simulink model "quad"  (R2018b)
settings: Solver=VariableStepAuto  StartTime=0.0  StopTime=100  RelTol=1e-3  EnableMultiTasking=on
InitFcn:
  | %%Motor
  | fs_servo = 50; %Hz
  | Ts_servo = 1/fs_servo;
  | rate = 1200; % rad/s per second change
  | limit = 1200; % rad/s
  | 
  | %%Controller
  | fs = 200; % Hz
  | Ts = 1/fs;
  | 
  | g = 9.81; % Gravity
values from neighbouring files (symbols this model uses):
  F = zeros(3, numPoints)    [test_cyclorotor.m]
  r = 0.069    [Cyclorotor.m]
undefined symbols (not defined in the file or in its folder): MIL
libraries: simulink x13, aerolibwind2 x1, sharedtransform x1
settings Model: Creator=fs349  LastModifiedBy=Jamie
settings DataIOCC: SaveState=on
settings OptimizationCC: LifeSpan=inf
settings DebuggingCC: AllowSymbolicDim=off  SFUnexpectedBacktrackingDiag=warning  SFNoUnconditionalDefaultTransitionDiag=warning  SFExecutionAtInitializationDiag=none
settings ModelReferenceCC: PropagateSignalLabelsOutOfModel=off
settings SFSimCC: SimUseLocalCustomCode=off
settings RTWCC: RTWUseLocalCustomCode=off
settings CodeAppCC: StateflowObjectComments=on
settings GRTTargetCC: TargetLangStandard=C89/C90 (ANSI)
settings ConfigComp: CovMetricSettings=dw  CovHtmlReporting=on  CovSaveCumulativeToWorkspaceVar=on  CovSaveSingleToWorkspaceVar=on  CovExternalEMLEnable=off

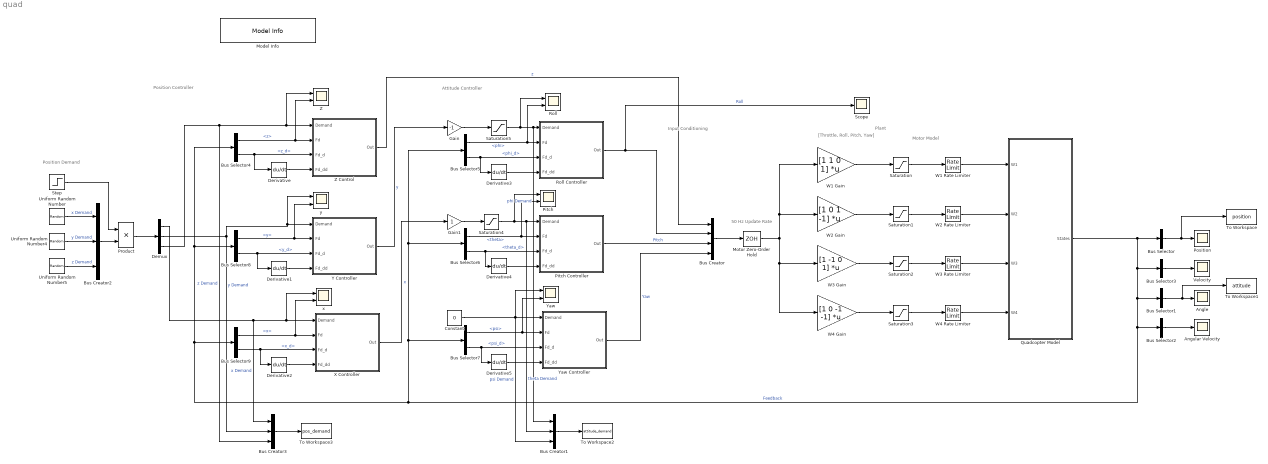
== system quad ==
  note: 50 Hz Update Rate
  note: Position Controller
  note: Attitude Controller
  note: Motor Model
  note: Plant
  note: Input Conditioning
  note: [Throttle, Roll, Pitch, Yaw]
  note: Position Demand
  Angle : Scope
  Angular Velocity : Scope
  Bus Creator : BusCreator  Inputs=4
  Bus Creator1 : BusCreator  Inputs=3
  Bus Creator2 : BusCreator  Inputs=3
  Bus Creator3 : BusCreator  Inputs=3
  Bus Selector : BusSelector  OutputSignals=x,y,z  OutputAsBus=on
  Bus Selector1 : BusSelector  OutputSignals=phi,theta,psi  OutputAsBus=on
  Bus Selector2 : BusSelector  OutputSignals=phi_d,theta_d,psi_d  OutputAsBus=on
  Bus Selector3 : BusSelector  OutputSignals=x_d,y_d,z_d  OutputAsBus=on
  Bus Selector4 : BusSelector  OutputSignals=z,z_d
  Bus Selector5 : BusSelector  OutputSignals=phi,phi_d
  Bus Selector6 : BusSelector  OutputSignals=theta,theta_d
  Bus Selector7 : BusSelector  OutputSignals=psi,psi_d
  Bus Selector8 : BusSelector  OutputSignals=y,y_d
  Bus Selector9 : BusSelector  OutputSignals=x,x_d
  Constant : Constant  Value=0
  Demux : Demux  Outputs=3
  Derivative{,1..5} (6 alike) : Derivative
  Gain : Gain  Gain=-1
  Gain1 : Gain
  Model Info : simulink/Model-Wide Utilities/Model Info  Frame=on  DisplayStringWithTags=|  HorizontalTextAlignment=Left  LeftAlignmentValue=0.02
      | Last Modified: %<ModifiedDate>
      | By: %<LastModifiedBy>
      | version: %<ModelVersion>
  Motor Zero-Order Hold : ZeroOrderHold  SampleTime=Ts_servo
  Pitch : Scope  NumInputPorts=2
  Pitch Controller : Subsystem  mask{P1=6, I1=0, D1=5, P2=1, I2=0, D2=0.03}
      mask prompts: P1 "P1, Proportional"; I1 "I1, Integral"; D1 "D1, Derivative"; P2 "P2, Proportional"; I2 "I2, Integral"; D2 "D2, Derivative"
      mask DialogControl Container3 Prompt: Outer Loop
      mask DialogControl Container4 Prompt: Inner Loop
  Position : Scope
  Product : Product
  Quadcopter Model : Subsystem  mask{g=g, m=0.468, k=2.98e-6, Ixx=4.856e-3, Iyy=4.856e-3, Izz=8.801e-3, b=1.14e-7, L=0.225, Ax=0.25, Ay=0.25, Az=0.25, ws=4.5}
      mask prompts: g "g, Gravity (m/s^2)"; m "m, Quad mass (kg)"; k "k, Angular velocity thrust proportional constant"; Ixx "Ixx, x inertia (kg m^2)"; Iyy "Iyy, y inertia (kg m^2)"; Izz "Izz, z intertia (kg m^2)"; b "b, Yaw torque angular velocity proportional constant"; L "L, Arm length (m)"; Ax "Ax, x drag Coefficient"; Ay "Ay, y drag Coefficien"; Az "Az, z drag Coefficien"; ws "ws, Wind Speed"
      mask DialogControl Container4 Prompt: Quad Properties
      mask DialogControl Container5 Prompt: Modelling Properies
  Roll : Scope  NumInputPorts=2
  Roll Controller : Subsystem  mask{P1=6, I1=0, D1=5, P2=1, I2=0, D2=0.03}
      mask prompts: P1 "P1, Proportional"; I1 "I1, Integral"; D1 "D1, Derivative"; P2 "P2, Proportional"; I2 "I2, Integral"; D2 "D2, Derivative"
      mask DialogControl Container3 Prompt: Outer Loop
      mask DialogControl Container4 Prompt: Inner Loop
  Saturation{,1..3} (4 alike) : Saturate  UpperLimit=limit  LowerLimit=0
  Saturation4 : Saturate  UpperLimit=pi/3  LowerLimit=-pi/3
  Saturation5 : Saturate  UpperLimit=pi/3  LowerLimit=-pi/3
  Scope : Scope
  Step : Step  Time=20  SampleTime=0
  To Workspace : ToWorkspace  VariableName=position  SaveFormat=Timeseries  SampleTime=-1
  To Workspace1 : ToWorkspace  VariableName=attitude  SaveFormat=Timeseries  SampleTime=-1
  To Workspace2 : ToWorkspace  VariableName=attitude_demand  SaveFormat=Timeseries  SampleTime=-1
  To Workspace3 : ToWorkspace  VariableName=pos_demand  SaveFormat=Timeseries  SampleTime=-1
  Uniform Random Number : UniformRandomNumber  Minimum=-3  Maximum=3  SampleTime=10
  Uniform Random Number4 : UniformRandomNumber  Minimum=-3  Maximum=3  Seed=1  SampleTime=10
  Uniform Random Number5 : UniformRandomNumber  Minimum=-3  Maximum=3  Seed=2  SampleTime=10
  Velocity : Scope
  W1 Gain : Gain  Gain=[1 1 0 1]  Multiplication=Matrix(K*u)
  W1 Rate Limiter : RateLimiter  RisingSlewLimit=rate  FallingSlewLimit=-rate
  W2 Gain : Gain  Gain=[1 0 1 -1]  Multiplication=Matrix(K*u)
  W2 Rate Limiter : RateLimiter  RisingSlewLimit=rate  FallingSlewLimit=-rate
  W3 Gain : Gain  Gain=[1 -1 0 1]  Multiplication=Matrix(K*u)
  W3 Rate Limiter : RateLimiter  RisingSlewLimit=rate  FallingSlewLimit=-rate
  W4 Gain : Gain  Gain=[1 0 -1 -1]  Multiplication=Matrix(K*u)
  W4 Rate Limiter : RateLimiter  RisingSlewLimit=rate  FallingSlewLimit=-rate
  X Controller : Subsystem  mask{P1=0.15, I1=0, D1=0.32, P2=0.6, I2=0, D2=0.18}
      mask prompts: P1 "P1, Proportional"; I1 "I1, Integral"; D1 "D1, Derivative"; P2 "P2, Proportional"; I2 "I2, Integral"; D2 "D2, Derivative"
      mask DialogControl Container3 Prompt: Outer Loop
      mask DialogControl Container4 Prompt: Inner Loop
  Y Controller : Subsystem  mask{P1=0.15, I1=0, D1=0.32, P2=0.6, I2=0, D2=0.18}
      mask prompts: P1 "P1, Proportional"; I1 "I1, Integral"; D1 "D1, Derivative"; P2 "P2, Proportional"; I2 "I2, Integral"; D2 "D2, Derivative"
      mask DialogControl Container3 Prompt: Outer Loop
      mask DialogControl Container4 Prompt: Inner Loop
  Yaw : Scope  NumInputPorts=2
  Yaw Controller : Subsystem  mask{P1=9, I1=0, D1=8, P2=6, I2=0, D2=1}
      mask prompts: P1 "P1, Proportional"; I1 "I1, Integral"; D1 "D1, Derivative"; P2 "P2, Proportional"; I2 "I2, Integral"; D2 "D2, Derivative"
      mask DialogControl Container3 Prompt: Outer Loop
      mask DialogControl Container4 Prompt: Inner Loop
  Z : Scope  NumInputPorts=2
  Z Control : Subsystem  mask{P1=12, I1=0, D1=15, P2=10, I2=4, D2=15}
      mask prompts: P1 "P1, Proportional"; I1 "I1, Integral"; D1 "D1, Derivative"; P2 "P2, Proportional"; I2 "I2, Integral"; D2 "D2, Derivative"
      mask DialogControl Container3 Prompt: Outer Loop
      mask DialogControl Container4 Prompt: Inner Loop
  x : Scope  NumInputPorts=2
  y : Scope  NumInputPorts=2
  wires:
  Bus Selector/1 -> Position/1, To Workspace/1
  Bus Selector1/1 -> Angle/1, To Workspace1/1
  Bus Selector2/1 -> Angular Velocity/1
  Bus Selector3/1 -> Velocity/1
  W1 Rate Limiter/1 -> Quadcopter Model/1(W1)
  W2 Rate Limiter/1 -> Quadcopter Model/2(W2)
  W3 Rate Limiter/1 -> Quadcopter Model/3(W3)
  W4 Rate Limiter/1 -> Quadcopter Model/4(W4)
  W1 Gain/1 -> Saturation/1
  W2 Gain/1 -> Saturation1/1
  W3 Gain/1 -> Saturation2/1
  W4 Gain/1 -> Saturation3/1
  Motor Zero-Order Hold/1 -> W1 Gain/1, W2 Gain/1, W4 Gain/1, W3 Gain/1
  Bus Creator/1 -> Motor Zero-Order Hold/1
  Roll Controller/1(Out) -> Scope/1, Bus Creator/2  "Roll"
  Z Control/1(Out) -> Bus Creator/1  "z"
  Bus Selector4/1 -> Z Control/2(Fd), Z/2  "<z>"
  Bus Selector4/2 -> Derivative/1, Z Control/3(Fd_d)  "<z_d>"
  Demux/3 -> Bus Creator3/3, Z/1, Z Control/1(Demand)  "z Demand"
  Saturation/1 -> W1 Rate Limiter/1
  Saturation1/1 -> W2 Rate Limiter/1
  Saturation2/1 -> W3 Rate Limiter/1
  Saturation3/1 -> W4 Rate Limiter/1
  Yaw Controller/1(Out) -> Bus Creator/4  "Yaw"
  Bus Selector5/1 -> Roll/2, Roll Controller/2(Fd)  "<phi>"
  Bus Selector5/2 -> Derivative3/1, Roll Controller/3(Fd_d)  "<phi_d>"
  Bus Selector6/2 -> Derivative4/1, Pitch Controller/3(Fd_d)  "<theta_d>"
  Bus Selector6/1 -> Pitch Controller/2(Fd), Pitch/2  "<theta>"
  Pitch Controller/1(Out) -> Bus Creator/3  "Pitch"
  Bus Selector7/1 -> Yaw Controller/2(Fd), Yaw/2  "<psi>"
  Bus Selector7/2 -> Derivative5/1, Yaw Controller/3(Fd_d)  "<psi_d>"
  Saturation4/1 -> Bus Creator1/2, Pitch Controller/1(Demand), Pitch/1  "theta Demand"
  Y Controller/1(Out) -> Gain/1  "y"
  Constant/1 -> Yaw/1, Bus Creator1/3, Yaw Controller/1(Demand)  "psi Demand"
  Quadcopter Model/1(States) -> Bus Selector/1, Bus Selector3/1, Bus Selector1/1, Bus Selector2/1, Bus Selector8/1, Bus Selector4/1, Bus Selector9/1, Bus Selector7/1, Bus Selector6/1, Bus Selector5/1  "Feedback"
  Bus Selector8/2 -> Derivative1/1, Y Controller/3(Fd_d)  "<y_d>"
  Bus Selector8/1 -> Y Controller/2(Fd), y/2  "<y>"
  Bus Selector9/1 -> x/2, X Controller/2(Fd)  "<x>"
  Bus Selector9/2 -> Derivative2/1, X Controller/3(Fd_d)  "<x_d>"
  Demux/2 -> y/1, Y Controller/1(Demand), Bus Creator3/2  "y Demand"
  Demux/1 -> x/1, X Controller/1(Demand), Bus Creator3/1  "x Demand"
  Saturation5/1 -> Roll/1, Bus Creator1/1, Roll Controller/1(Demand)  "phi Demand"
  X Controller/1(Out) -> Gain1/1  "x"
  Gain/1 -> Saturation5/1
  Gain1/1 -> Saturation4/1
  Derivative/1 -> Z Control/4(Fd_dd)
  Derivative1/1 -> Y Controller/4(Fd_dd)
  Derivative2/1 -> X Controller/4(Fd_dd)
  Derivative5/1 -> Yaw Controller/4(Fd_dd)
  Derivative4/1 -> Pitch Controller/4(Fd_dd)
  Derivative3/1 -> Roll Controller/4(Fd_dd)
  Uniform Random Number5/1 -> Bus Creator2/3  "z Demand"
  Uniform Random Number4/1 -> Bus Creator2/2  "y Demand"
  Uniform Random Number/1 -> Bus Creator2/1  "x Demand"
  Bus Creator2/1 -> Product/2
  Step/1 -> Product/1
  Product/1 -> Demux/1
  Bus Creator1/1 -> To Workspace2/1
  Bus Creator3/1 -> To Workspace3/1

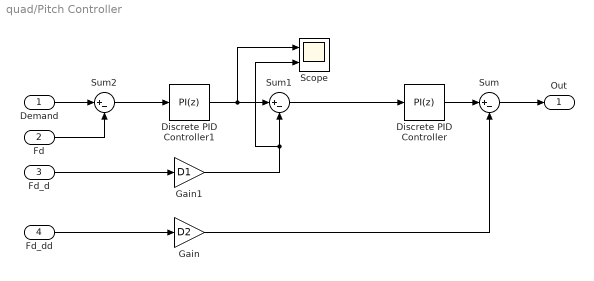
== system quad/Pitch Controller ==
  Demand : Inport
  Fd : Inport  Port=2
  Fd_d : Inport  Port=3
  Fd_dd : Inport  Port=4
  Discrete PID Controller : simulink/Continuous/PID Controller  Controller=PI  Form=Parallel  TimeDomain=Discrete-time  SampleTime=Ts  IntegratorMethod=Forward Euler  FilterMethod=Forward Euler  ControllerParametersSource=internal  P=P2  I=I2  D=0  UseFilter=off  N=100  TunerSelectOption=Transfer Function Based (PID Tuner App)  InitialConditionSource=internal  InitialConditionForIntegrator=0  InitialConditionForFilter=0  DifferentiatorICPrevScaledInput=0  ExternalReset=none  TrackingMode=off  Kt=1  LimitOutput=off  UpperSaturationLimit=inf  LowerSaturationLimit=-inf  LinearizeAsGain=off  AntiWindupMode=none  Kb=1  POutMin=[]  POutMax=[]  IOutMin=[]  IOutMax=[]  DOutMin=[]  DOutMax=[]  NOutMin=[]  NOutMax=[]  SumOutMin=[]  SumOutMax=[]  SaturationOutMin=[]  SaturationOutMax=[]  PParamMin=[]  PParamMax=[]  IParamMin=[]  IParamMax=[]  DParamMin=[]  DParamMax=[]  NParamMin=[]  NParamMax=[]  KbParamMin=[]  KbParamMax=[]  KtParamMin=[]  KtParamMax=[]  KbOutMin=[]  KbOutMax=[]  KtOutMin=[]  KtOutMax=[]  IntegratorOutMin=[]  IntegratorOutMax=[]  FilterOutMin=[]  FilterOutMax=[]  SumI1OutMin=[]  SumI1OutMax=[]  SumI2OutMin=[]  SumI2OutMax=[]  SumI3OutMin=[]  SumI3OutMax=[]  SumI4OutMin=[]  SumI4OutMax=[]  SumDOutMin=[]  SumDOutMax=[]  DifferentiatorOutMin=[]  DifferentiatorOutMax=[]  FilterDiffOutCoefMin=[]  FilterDiffOutCoefMax=[]  ReciprocalOutMin=[]  ReciprocalOutMax=[]  SumDenOutMin=[]  SumDenOutMax=[]  SumNumOutMin=[]  SumNumOutMax=[]  DivideOutMin=[]  DivideOutMax=[]  IntegratorContinuousStateAttributes=''  IntegratorStateMustResolveToSignalObject=off  IntegratorRTWStateStorageClass=Auto  FilterContinuousStateAttributes=''  FilterStateMustResolveToSignalObject=off  FilterRTWStateStorageClass=Auto  ParallelPVariant=InternalParameters  IdealPVariant=Disabled  IVariant=InternalParameters  DVariant=Disabled  IntegratorVariant=Discrete  SatVariant=Disabled  AWVariant=Passthrough  PCopyVariant=Disabled  TRVariant=Disabled  FdbkBlocksVariant=Forward  IdealPFdbkVariant=Disabled  SatFdbkVariant=Disabled  DerivativeFilterVariant=Disabled  NVariant=Disabled  NCopyVariant=Disabled_SignalSpec  FilterICVariant=Disabled  IntegratorICVariant=InternalICs  ExternalResetVariant=Disabled  TRSumVariant=Passthrough  SumFdbkVariant=Disabled  SumVariant=Sum_PI
  Discrete PID Controller1 : simulink/Continuous/PID Controller  Controller=PI  Form=Parallel  TimeDomain=Discrete-time  SampleTime=Ts  IntegratorMethod=Forward Euler  FilterMethod=Forward Euler  ControllerParametersSource=internal  P=P1  I=I1  D=0  UseFilter=off  N=100  TunerSelectOption=Transfer Function Based (PID Tuner App)  InitialConditionSource=internal  InitialConditionForIntegrator=0  InitialConditionForFilter=0  DifferentiatorICPrevScaledInput=0  ExternalReset=none  TrackingMode=off  Kt=1  LimitOutput=off  UpperSaturationLimit=inf  LowerSaturationLimit=-inf  LinearizeAsGain=off  AntiWindupMode=none  Kb=1  POutMin=[]  POutMax=[]  IOutMin=[]  IOutMax=[]  DOutMin=[]  DOutMax=[]  NOutMin=[]  NOutMax=[]  SumOutMin=[]  SumOutMax=[]  SaturationOutMin=[]  SaturationOutMax=[]  PParamMin=[]  PParamMax=[]  IParamMin=[]  IParamMax=[]  DParamMin=[]  DParamMax=[]  NParamMin=[]  NParamMax=[]  KbParamMin=[]  KbParamMax=[]  KtParamMin=[]  KtParamMax=[]  KbOutMin=[]  KbOutMax=[]  KtOutMin=[]  KtOutMax=[]  IntegratorOutMin=[]  IntegratorOutMax=[]  FilterOutMin=[]  FilterOutMax=[]  SumI1OutMin=[]  SumI1OutMax=[]  SumI2OutMin=[]  SumI2OutMax=[]  SumI3OutMin=[]  SumI3OutMax=[]  SumI4OutMin=[]  SumI4OutMax=[]  SumDOutMin=[]  SumDOutMax=[]  DifferentiatorOutMin=[]  DifferentiatorOutMax=[]  FilterDiffOutCoefMin=[]  FilterDiffOutCoefMax=[]  ReciprocalOutMin=[]  ReciprocalOutMax=[]  SumDenOutMin=[]  SumDenOutMax=[]  SumNumOutMin=[]  SumNumOutMax=[]  DivideOutMin=[]  DivideOutMax=[]  IntegratorContinuousStateAttributes=''  IntegratorStateMustResolveToSignalObject=off  IntegratorRTWStateStorageClass=Auto  FilterContinuousStateAttributes=''  FilterStateMustResolveToSignalObject=off  FilterRTWStateStorageClass=Auto  ParallelPVariant=InternalParameters  IdealPVariant=Disabled  IVariant=InternalParameters  DVariant=Disabled  IntegratorVariant=Discrete  SatVariant=Disabled  AWVariant=Passthrough  PCopyVariant=Disabled  TRVariant=Disabled  FdbkBlocksVariant=Forward  IdealPFdbkVariant=Disabled  SatFdbkVariant=Disabled  DerivativeFilterVariant=Disabled  NVariant=Disabled  NCopyVariant=Disabled_SignalSpec  FilterICVariant=Disabled  IntegratorICVariant=InternalICs  ExternalResetVariant=Disabled  TRSumVariant=Passthrough  SumFdbkVariant=Disabled  SumVariant=Sum_PI
  Gain : Gain  Gain=D2
  Gain1 : Gain  Gain=D1
  Scope : Scope  NumInputPorts=2
  Sum : Sum  Inputs=|+-
  Sum1 : Sum  Inputs=|+-
  Sum2 : Sum  Inputs=|+-
  Out : Outport
  wires:
  Sum1/1 -> Discrete PID Controller/1
  Gain1/1 -> Scope/2, Sum1/2
  Discrete PID Controller/1 -> Sum/1
  Sum/1 -> Out/1
  Fd_dd/1 -> Gain/1
  Sum2/1 -> Discrete PID Controller1/1
  Gain/1 -> Sum/2
  Fd/1 -> Sum2/2
  Fd_d/1 -> Gain1/1
  Demand/1 -> Sum2/1
  Discrete PID Controller1/1 -> Scope/1, Sum1/1

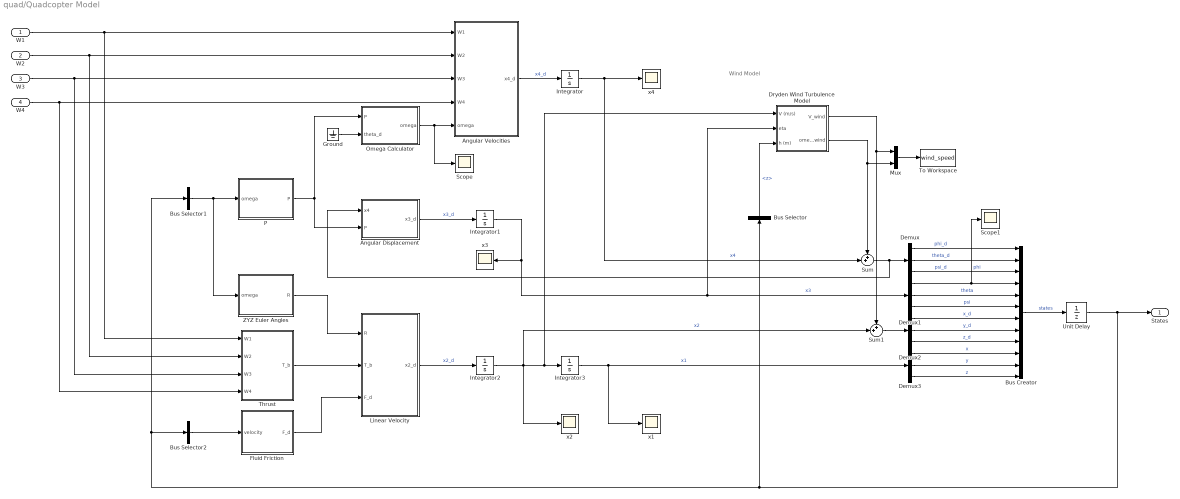
== system quad/Quadcopter Model ==
  note: Wind Model
  W1 : Inport
  W2 : Inport  Port=2
  W3 : Inport  Port=3
  W4 : Inport  Port=4
  Angular Displacement : MATLAB Function  TreatAsAtomicUnit=on
  Angular Velocities : MATLAB Function  TreatAsAtomicUnit=on  mask{Ixx=Ixx, Iyy=Iyy, Izz=Izz, k=k, b=b, L=L}
      mask prompts: k "k, motor speed to torque constant"
  Bus Creator : BusCreator  Inputs=12
  Bus Selector : BusSelector  OutputSignals=z
  Bus Selector1 : BusSelector  OutputSignals=phi,theta,psi  OutputAsBus=on
  Bus Selector2 : BusSelector  OutputSignals=x_d,y_d,z_d  OutputAsBus=on
  Demux{,1..3} (4 alike) : Demux  Outputs=3
  Dryden Wind Turbulence Model : Subsystem  mask{ws=ws}
      mask prompts: ws "ws, wind speed (m/s)"
  Fluid Friction : MATLAB Function  TreatAsAtomicUnit=on  mask{Ax=Ax, Ay=Ay, Az=Az}
      mask prompts: Ax "Ax, x Drag Coefficient"; Ay "Ay, y Drag coefficient"; Az "Az, z Drag Coefficient"
  Ground : Ground
  Integrator{,1..3} (4 alike) : Integrator
  Linear Velocity : MATLAB Function  TreatAsAtomicUnit=on  mask{g=g, m=m}
      mask prompts: g "g, Gravity"; m "m, mass"
  Mux : Mux  Inputs=2
  Omega Calculator : MATLAB Function  TreatAsAtomicUnit=on
  P : MATLAB Function  TreatAsAtomicUnit=on
  Scope : Scope
  Scope1 : Scope
  Sum : Sum  Inputs=++|
  Sum1 : Sum  Inputs=++|
  Thrust : MATLAB Function  TreatAsAtomicUnit=on  mask{k=k}
  To Workspace : ToWorkspace  VariableName=wind_speed  SaveFormat=Timeseries  SampleTime=-1
  Unit Delay : UnitDelay  SampleTime=Ts
  ZYZ Euler Angles : MATLAB Function  TreatAsAtomicUnit=on
  x{1..4} (4 alike) : Scope
  States : Outport
  wires:
  Integrator1/1 -> x3/1, Dryden Wind Turbulence Model/2(eta), Demux1/1  "x3"
  ZYZ Euler Angles/1(R) -> Linear Velocity/1(R)
  Angular Displacement/1(x3_d) -> Integrator1/1  "x3_d"
  Integrator/1 -> x4/1, Sum/2  "x4"
  Fluid Friction/1(F_d) -> Linear Velocity/3(F_d)
  Thrust/1(T_b) -> Linear Velocity/2(T_b)
  Integrator2/1 -> Sum1/2, x2/1, Dryden Wind Turbulence Model/1(V (m/s)), Integrator3/1  "x2"
  Linear Velocity/1(x2_d) -> Integrator2/1  "x2_d"
  Bus Creator/1 -> Unit Delay/1  "states"
  Integrator3/1 -> x1/1, Demux3/1  "x1"
  W1/1 -> Angular Velocities/1(W1), Thrust/1(W1)
  W4/1 -> Angular Velocities/4(W4), Thrust/4(W4)
  W2/1 -> Angular Velocities/2(W2), Thrust/2(W2)
  W3/1 -> Angular Velocities/3(W3), Thrust/3(W3)
  P/1(P) -> Omega Calculator/1(P), Angular Displacement/2(P)
  Omega Calculator/1(omega) -> Scope/1, Angular Velocities/5(omega)
  Angular Velocities/1(x4_d) -> Integrator/1  "x4_d"
  Bus Selector1/1 -> ZYZ Euler Angles/1(omega), P/1(omega)
  Bus Selector2/1 -> Fluid Friction/1(velocity)
  Demux3/3 -> Bus Creator/12  "z"
  Demux/2 -> Bus Creator/2  "theta_d"
  Demux3/2 -> Bus Creator/11  "y"
  Demux3/1 -> Bus Creator/10  "x"
  Demux2/3 -> Bus Creator/9  "z_d"
  Demux2/2 -> Bus Creator/8  "y_d"
  Demux2/1 -> Bus Creator/7  "x_d"
  Demux/1 -> Bus Creator/1  "phi_d"
  Demux1/3 -> Bus Creator/6  "psi"
  Demux1/2 -> Bus Creator/5  "theta"
  Demux1/1 -> Scope1/1, Bus Creator/4  "phi"
  Demux/3 -> Bus Creator/3  "psi_d"
  Unit Delay/1 -> States/1, Bus Selector/1, Bus Selector1/1, Bus Selector2/1
  Bus Selector/1 -> Dryden Wind Turbulence Model/3(h (m))  "<z>"
  Dryden Wind Turbulence Model/2(omega_wind) -> Mux/2, Sum/1
  Dryden Wind Turbulence Model/1(V_wind) -> Mux/1, Sum1/1
  Sum/1 -> Angular Displacement/1(x4), Demux/1
  Sum1/1 -> Demux2/1
  Ground/1 -> Omega Calculator/2(theta_d)
  Mux/1 -> To Workspace/1

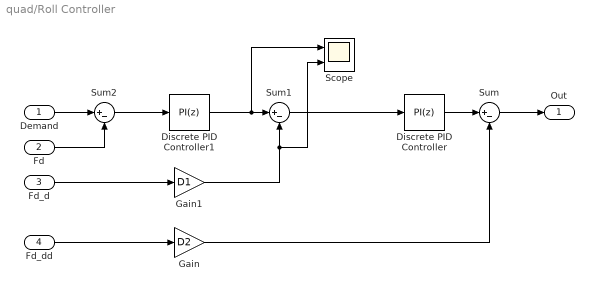
== system quad/Roll Controller ==
  Demand : Inport
  Fd : Inport  Port=2
  Fd_d : Inport  Port=3
  Fd_dd : Inport  Port=4
  Discrete PID Controller : simulink/Continuous/PID Controller  Controller=PI  Form=Parallel  TimeDomain=Discrete-time  SampleTime=Ts  IntegratorMethod=Forward Euler  FilterMethod=Forward Euler  ControllerParametersSource=internal  P=P2  I=I2  D=0  UseFilter=off  N=100  TunerSelectOption=Transfer Function Based (PID Tuner App)  InitialConditionSource=internal  InitialConditionForIntegrator=0  InitialConditionForFilter=0  DifferentiatorICPrevScaledInput=0  ExternalReset=none  TrackingMode=off  Kt=1  LimitOutput=off  UpperSaturationLimit=inf  LowerSaturationLimit=-inf  LinearizeAsGain=off  AntiWindupMode=none  Kb=1  POutMin=[]  POutMax=[]  IOutMin=[]  IOutMax=[]  DOutMin=[]  DOutMax=[]  NOutMin=[]  NOutMax=[]  SumOutMin=[]  SumOutMax=[]  SaturationOutMin=[]  SaturationOutMax=[]  PParamMin=[]  PParamMax=[]  IParamMin=[]  IParamMax=[]  DParamMin=[]  DParamMax=[]  NParamMin=[]  NParamMax=[]  KbParamMin=[]  KbParamMax=[]  KtParamMin=[]  KtParamMax=[]  KbOutMin=[]  KbOutMax=[]  KtOutMin=[]  KtOutMax=[]  IntegratorOutMin=[]  IntegratorOutMax=[]  FilterOutMin=[]  FilterOutMax=[]  SumI1OutMin=[]  SumI1OutMax=[]  SumI2OutMin=[]  SumI2OutMax=[]  SumI3OutMin=[]  SumI3OutMax=[]  SumI4OutMin=[]  SumI4OutMax=[]  SumDOutMin=[]  SumDOutMax=[]  DifferentiatorOutMin=[]  DifferentiatorOutMax=[]  FilterDiffOutCoefMin=[]  FilterDiffOutCoefMax=[]  ReciprocalOutMin=[]  ReciprocalOutMax=[]  SumDenOutMin=[]  SumDenOutMax=[]  SumNumOutMin=[]  SumNumOutMax=[]  DivideOutMin=[]  DivideOutMax=[]  IntegratorContinuousStateAttributes=''  IntegratorStateMustResolveToSignalObject=off  IntegratorRTWStateStorageClass=Auto  FilterContinuousStateAttributes=''  FilterStateMustResolveToSignalObject=off  FilterRTWStateStorageClass=Auto  ParallelPVariant=InternalParameters  IdealPVariant=Disabled  IVariant=InternalParameters  DVariant=Disabled  IntegratorVariant=Discrete  SatVariant=Disabled  AWVariant=Passthrough  PCopyVariant=Disabled  TRVariant=Disabled  FdbkBlocksVariant=Forward  IdealPFdbkVariant=Disabled  SatFdbkVariant=Disabled  DerivativeFilterVariant=Disabled  NVariant=Disabled  NCopyVariant=Disabled_SignalSpec  FilterICVariant=Disabled  IntegratorICVariant=InternalICs  ExternalResetVariant=Disabled  TRSumVariant=Passthrough  SumFdbkVariant=Disabled  SumVariant=Sum_PI
  Discrete PID Controller1 : simulink/Continuous/PID Controller  Controller=PI  Form=Parallel  TimeDomain=Discrete-time  SampleTime=Ts  IntegratorMethod=Forward Euler  FilterMethod=Forward Euler  ControllerParametersSource=internal  P=P1  I=I1  D=0  UseFilter=off  N=100  TunerSelectOption=Transfer Function Based (PID Tuner App)  InitialConditionSource=internal  InitialConditionForIntegrator=0  InitialConditionForFilter=0  DifferentiatorICPrevScaledInput=0  ExternalReset=none  TrackingMode=off  Kt=1  LimitOutput=off  UpperSaturationLimit=inf  LowerSaturationLimit=-inf  LinearizeAsGain=off  AntiWindupMode=none  Kb=1  POutMin=[]  POutMax=[]  IOutMin=[]  IOutMax=[]  DOutMin=[]  DOutMax=[]  NOutMin=[]  NOutMax=[]  SumOutMin=[]  SumOutMax=[]  SaturationOutMin=[]  SaturationOutMax=[]  PParamMin=[]  PParamMax=[]  IParamMin=[]  IParamMax=[]  DParamMin=[]  DParamMax=[]  NParamMin=[]  NParamMax=[]  KbParamMin=[]  KbParamMax=[]  KtParamMin=[]  KtParamMax=[]  KbOutMin=[]  KbOutMax=[]  KtOutMin=[]  KtOutMax=[]  IntegratorOutMin=[]  IntegratorOutMax=[]  FilterOutMin=[]  FilterOutMax=[]  SumI1OutMin=[]  SumI1OutMax=[]  SumI2OutMin=[]  SumI2OutMax=[]  SumI3OutMin=[]  SumI3OutMax=[]  SumI4OutMin=[]  SumI4OutMax=[]  SumDOutMin=[]  SumDOutMax=[]  DifferentiatorOutMin=[]  DifferentiatorOutMax=[]  FilterDiffOutCoefMin=[]  FilterDiffOutCoefMax=[]  ReciprocalOutMin=[]  ReciprocalOutMax=[]  SumDenOutMin=[]  SumDenOutMax=[]  SumNumOutMin=[]  SumNumOutMax=[]  DivideOutMin=[]  DivideOutMax=[]  IntegratorContinuousStateAttributes=''  IntegratorStateMustResolveToSignalObject=off  IntegratorRTWStateStorageClass=Auto  FilterContinuousStateAttributes=''  FilterStateMustResolveToSignalObject=off  FilterRTWStateStorageClass=Auto  ParallelPVariant=InternalParameters  IdealPVariant=Disabled  IVariant=InternalParameters  DVariant=Disabled  IntegratorVariant=Discrete  SatVariant=Disabled  AWVariant=Passthrough  PCopyVariant=Disabled  TRVariant=Disabled  FdbkBlocksVariant=Forward  IdealPFdbkVariant=Disabled  SatFdbkVariant=Disabled  DerivativeFilterVariant=Disabled  NVariant=Disabled  NCopyVariant=Disabled_SignalSpec  FilterICVariant=Disabled  IntegratorICVariant=InternalICs  ExternalResetVariant=Disabled  TRSumVariant=Passthrough  SumFdbkVariant=Disabled  SumVariant=Sum_PI
  Gain : Gain  Gain=D2
  Gain1 : Gain  Gain=D1
  Scope : Scope  NumInputPorts=2
  Sum : Sum  Inputs=|+-
  Sum1 : Sum  Inputs=|+-
  Sum2 : Sum  Inputs=|+-
  Out : Outport
  wires:
  Demand/1 -> Sum2/1
  Discrete PID Controller1/1 -> Scope/1, Sum1/1
  Fd_d/1 -> Gain1/1
  Fd/1 -> Sum2/2
  Gain/1 -> Sum/2
  Sum2/1 -> Discrete PID Controller1/1
  Fd_dd/1 -> Gain/1
  Sum/1 -> Out/1
  Discrete PID Controller/1 -> Sum/1
  Sum1/1 -> Discrete PID Controller/1
  Gain1/1 -> Scope/2, Sum1/2

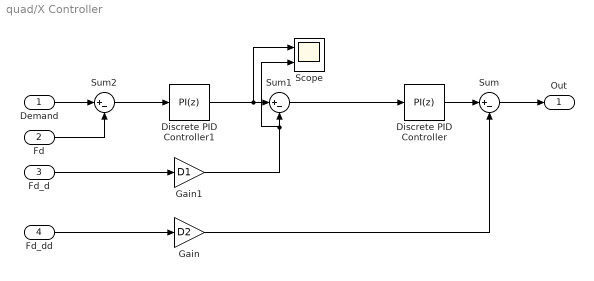
== system quad/X Controller ==
  Demand : Inport
  Fd : Inport  Port=2
  Fd_d : Inport  Port=3
  Fd_dd : Inport  Port=4
  Discrete PID Controller : simulink/Continuous/PID Controller  Controller=PI  Form=Parallel  TimeDomain=Discrete-time  SampleTime=Ts  IntegratorMethod=Forward Euler  FilterMethod=Forward Euler  ControllerParametersSource=internal  P=P2  I=I2  D=0  UseFilter=off  N=100  TunerSelectOption=Transfer Function Based (PID Tuner App)  InitialConditionSource=internal  InitialConditionForIntegrator=0  InitialConditionForFilter=0  DifferentiatorICPrevScaledInput=0  ExternalReset=none  TrackingMode=off  Kt=1  LimitOutput=off  UpperSaturationLimit=inf  LowerSaturationLimit=-inf  LinearizeAsGain=off  AntiWindupMode=none  Kb=1  POutMin=[]  POutMax=[]  IOutMin=[]  IOutMax=[]  DOutMin=[]  DOutMax=[]  NOutMin=[]  NOutMax=[]  SumOutMin=[]  SumOutMax=[]  SaturationOutMin=[]  SaturationOutMax=[]  PParamMin=[]  PParamMax=[]  IParamMin=[]  IParamMax=[]  DParamMin=[]  DParamMax=[]  NParamMin=[]  NParamMax=[]  KbParamMin=[]  KbParamMax=[]  KtParamMin=[]  KtParamMax=[]  KbOutMin=[]  KbOutMax=[]  KtOutMin=[]  KtOutMax=[]  IntegratorOutMin=[]  IntegratorOutMax=[]  FilterOutMin=[]  FilterOutMax=[]  SumI1OutMin=[]  SumI1OutMax=[]  SumI2OutMin=[]  SumI2OutMax=[]  SumI3OutMin=[]  SumI3OutMax=[]  SumI4OutMin=[]  SumI4OutMax=[]  SumDOutMin=[]  SumDOutMax=[]  DifferentiatorOutMin=[]  DifferentiatorOutMax=[]  FilterDiffOutCoefMin=[]  FilterDiffOutCoefMax=[]  ReciprocalOutMin=[]  ReciprocalOutMax=[]  SumDenOutMin=[]  SumDenOutMax=[]  SumNumOutMin=[]  SumNumOutMax=[]  DivideOutMin=[]  DivideOutMax=[]  IntegratorContinuousStateAttributes=''  IntegratorStateMustResolveToSignalObject=off  IntegratorRTWStateStorageClass=Auto  FilterContinuousStateAttributes=''  FilterStateMustResolveToSignalObject=off  FilterRTWStateStorageClass=Auto  ParallelPVariant=InternalParameters  IdealPVariant=Disabled  IVariant=InternalParameters  DVariant=Disabled  IntegratorVariant=Discrete  SatVariant=Disabled  AWVariant=Passthrough  PCopyVariant=Disabled  TRVariant=Disabled  FdbkBlocksVariant=Forward  IdealPFdbkVariant=Disabled  SatFdbkVariant=Disabled  DerivativeFilterVariant=Disabled  NVariant=Disabled  NCopyVariant=Disabled_SignalSpec  FilterICVariant=Disabled  IntegratorICVariant=InternalICs  ExternalResetVariant=Disabled  TRSumVariant=Passthrough  SumFdbkVariant=Disabled  SumVariant=Sum_PI
  Discrete PID Controller1 : simulink/Continuous/PID Controller  Controller=PI  Form=Parallel  TimeDomain=Discrete-time  SampleTime=Ts  IntegratorMethod=Forward Euler  FilterMethod=Forward Euler  ControllerParametersSource=internal  P=P1  I=I1  D=0  UseFilter=off  N=100  TunerSelectOption=Transfer Function Based (PID Tuner App)  InitialConditionSource=internal  InitialConditionForIntegrator=0  InitialConditionForFilter=0  DifferentiatorICPrevScaledInput=0  ExternalReset=none  TrackingMode=off  Kt=1  LimitOutput=off  UpperSaturationLimit=inf  LowerSaturationLimit=-inf  LinearizeAsGain=off  AntiWindupMode=none  Kb=1  POutMin=[]  POutMax=[]  IOutMin=[]  IOutMax=[]  DOutMin=[]  DOutMax=[]  NOutMin=[]  NOutMax=[]  SumOutMin=[]  SumOutMax=[]  SaturationOutMin=[]  SaturationOutMax=[]  PParamMin=[]  PParamMax=[]  IParamMin=[]  IParamMax=[]  DParamMin=[]  DParamMax=[]  NParamMin=[]  NParamMax=[]  KbParamMin=[]  KbParamMax=[]  KtParamMin=[]  KtParamMax=[]  KbOutMin=[]  KbOutMax=[]  KtOutMin=[]  KtOutMax=[]  IntegratorOutMin=[]  IntegratorOutMax=[]  FilterOutMin=[]  FilterOutMax=[]  SumI1OutMin=[]  SumI1OutMax=[]  SumI2OutMin=[]  SumI2OutMax=[]  SumI3OutMin=[]  SumI3OutMax=[]  SumI4OutMin=[]  SumI4OutMax=[]  SumDOutMin=[]  SumDOutMax=[]  DifferentiatorOutMin=[]  DifferentiatorOutMax=[]  FilterDiffOutCoefMin=[]  FilterDiffOutCoefMax=[]  ReciprocalOutMin=[]  ReciprocalOutMax=[]  SumDenOutMin=[]  SumDenOutMax=[]  SumNumOutMin=[]  SumNumOutMax=[]  DivideOutMin=[]  DivideOutMax=[]  IntegratorContinuousStateAttributes=''  IntegratorStateMustResolveToSignalObject=off  IntegratorRTWStateStorageClass=Auto  FilterContinuousStateAttributes=''  FilterStateMustResolveToSignalObject=off  FilterRTWStateStorageClass=Auto  ParallelPVariant=InternalParameters  IdealPVariant=Disabled  IVariant=InternalParameters  DVariant=Disabled  IntegratorVariant=Discrete  SatVariant=Disabled  AWVariant=Passthrough  PCopyVariant=Disabled  TRVariant=Disabled  FdbkBlocksVariant=Forward  IdealPFdbkVariant=Disabled  SatFdbkVariant=Disabled  DerivativeFilterVariant=Disabled  NVariant=Disabled  NCopyVariant=Disabled_SignalSpec  FilterICVariant=Disabled  IntegratorICVariant=InternalICs  ExternalResetVariant=Disabled  TRSumVariant=Passthrough  SumFdbkVariant=Disabled  SumVariant=Sum_PI
  Gain : Gain  Gain=D2
  Gain1 : Gain  Gain=D1
  Scope : Scope  NumInputPorts=2
  Sum : Sum  Inputs=|+-
  Sum1 : Sum  Inputs=|+-
  Sum2 : Sum  Inputs=|+-
  Out : Outport
  wires:
  Demand/1 -> Sum2/1
  Discrete PID Controller1/1 -> Scope/1, Sum1/1
  Fd_d/1 -> Gain1/1
  Fd/1 -> Sum2/2
  Gain/1 -> Sum/2
  Sum2/1 -> Discrete PID Controller1/1
  Fd_dd/1 -> Gain/1
  Sum/1 -> Out/1
  Discrete PID Controller/1 -> Sum/1
  Sum1/1 -> Discrete PID Controller/1
  Gain1/1 -> Scope/2, Sum1/2

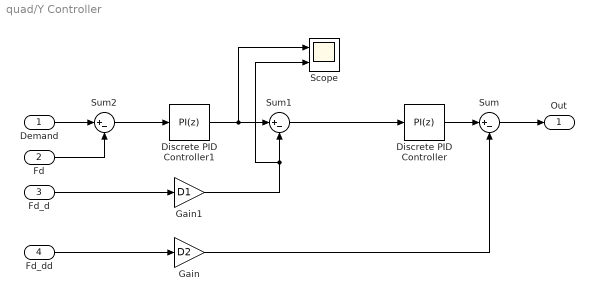
== system quad/Y Controller ==
  Demand : Inport
  Fd : Inport  Port=2
  Fd_d : Inport  Port=3
  Fd_dd : Inport  Port=4
  Discrete PID Controller : simulink/Continuous/PID Controller  Controller=PI  Form=Parallel  TimeDomain=Discrete-time  SampleTime=Ts  IntegratorMethod=Forward Euler  FilterMethod=Forward Euler  ControllerParametersSource=internal  P=P2  I=I2  D=0  UseFilter=off  N=100  TunerSelectOption=Transfer Function Based (PID Tuner App)  InitialConditionSource=internal  InitialConditionForIntegrator=0  InitialConditionForFilter=0  DifferentiatorICPrevScaledInput=0  ExternalReset=none  TrackingMode=off  Kt=1  LimitOutput=off  UpperSaturationLimit=inf  LowerSaturationLimit=-inf  LinearizeAsGain=off  AntiWindupMode=none  Kb=1  POutMin=[]  POutMax=[]  IOutMin=[]  IOutMax=[]  DOutMin=[]  DOutMax=[]  NOutMin=[]  NOutMax=[]  SumOutMin=[]  SumOutMax=[]  SaturationOutMin=[]  SaturationOutMax=[]  PParamMin=[]  PParamMax=[]  IParamMin=[]  IParamMax=[]  DParamMin=[]  DParamMax=[]  NParamMin=[]  NParamMax=[]  KbParamMin=[]  KbParamMax=[]  KtParamMin=[]  KtParamMax=[]  KbOutMin=[]  KbOutMax=[]  KtOutMin=[]  KtOutMax=[]  IntegratorOutMin=[]  IntegratorOutMax=[]  FilterOutMin=[]  FilterOutMax=[]  SumI1OutMin=[]  SumI1OutMax=[]  SumI2OutMin=[]  SumI2OutMax=[]  SumI3OutMin=[]  SumI3OutMax=[]  SumI4OutMin=[]  SumI4OutMax=[]  SumDOutMin=[]  SumDOutMax=[]  DifferentiatorOutMin=[]  DifferentiatorOutMax=[]  FilterDiffOutCoefMin=[]  FilterDiffOutCoefMax=[]  ReciprocalOutMin=[]  ReciprocalOutMax=[]  SumDenOutMin=[]  SumDenOutMax=[]  SumNumOutMin=[]  SumNumOutMax=[]  DivideOutMin=[]  DivideOutMax=[]  IntegratorContinuousStateAttributes=''  IntegratorStateMustResolveToSignalObject=off  IntegratorRTWStateStorageClass=Auto  FilterContinuousStateAttributes=''  FilterStateMustResolveToSignalObject=off  FilterRTWStateStorageClass=Auto  ParallelPVariant=InternalParameters  IdealPVariant=Disabled  IVariant=InternalParameters  DVariant=Disabled  IntegratorVariant=Discrete  SatVariant=Disabled  AWVariant=Passthrough  PCopyVariant=Disabled  TRVariant=Disabled  FdbkBlocksVariant=Forward  IdealPFdbkVariant=Disabled  SatFdbkVariant=Disabled  DerivativeFilterVariant=Disabled  NVariant=Disabled  NCopyVariant=Disabled_SignalSpec  FilterICVariant=Disabled  IntegratorICVariant=InternalICs  ExternalResetVariant=Disabled  TRSumVariant=Passthrough  SumFdbkVariant=Disabled  SumVariant=Sum_PI
  Discrete PID Controller1 : simulink/Continuous/PID Controller  Controller=PI  Form=Parallel  TimeDomain=Discrete-time  SampleTime=Ts  IntegratorMethod=Forward Euler  FilterMethod=Forward Euler  ControllerParametersSource=internal  P=P1  I=I1  D=0  UseFilter=off  N=100  TunerSelectOption=Transfer Function Based (PID Tuner App)  InitialConditionSource=internal  InitialConditionForIntegrator=0  InitialConditionForFilter=0  DifferentiatorICPrevScaledInput=0  ExternalReset=none  TrackingMode=off  Kt=1  LimitOutput=off  UpperSaturationLimit=inf  LowerSaturationLimit=-inf  LinearizeAsGain=off  AntiWindupMode=none  Kb=1  POutMin=[]  POutMax=[]  IOutMin=[]  IOutMax=[]  DOutMin=[]  DOutMax=[]  NOutMin=[]  NOutMax=[]  SumOutMin=[]  SumOutMax=[]  SaturationOutMin=[]  SaturationOutMax=[]  PParamMin=[]  PParamMax=[]  IParamMin=[]  IParamMax=[]  DParamMin=[]  DParamMax=[]  NParamMin=[]  NParamMax=[]  KbParamMin=[]  KbParamMax=[]  KtParamMin=[]  KtParamMax=[]  KbOutMin=[]  KbOutMax=[]  KtOutMin=[]  KtOutMax=[]  IntegratorOutMin=[]  IntegratorOutMax=[]  FilterOutMin=[]  FilterOutMax=[]  SumI1OutMin=[]  SumI1OutMax=[]  SumI2OutMin=[]  SumI2OutMax=[]  SumI3OutMin=[]  SumI3OutMax=[]  SumI4OutMin=[]  SumI4OutMax=[]  SumDOutMin=[]  SumDOutMax=[]  DifferentiatorOutMin=[]  DifferentiatorOutMax=[]  FilterDiffOutCoefMin=[]  FilterDiffOutCoefMax=[]  ReciprocalOutMin=[]  ReciprocalOutMax=[]  SumDenOutMin=[]  SumDenOutMax=[]  SumNumOutMin=[]  SumNumOutMax=[]  DivideOutMin=[]  DivideOutMax=[]  IntegratorContinuousStateAttributes=''  IntegratorStateMustResolveToSignalObject=off  IntegratorRTWStateStorageClass=Auto  FilterContinuousStateAttributes=''  FilterStateMustResolveToSignalObject=off  FilterRTWStateStorageClass=Auto  ParallelPVariant=InternalParameters  IdealPVariant=Disabled  IVariant=InternalParameters  DVariant=Disabled  IntegratorVariant=Discrete  SatVariant=Disabled  AWVariant=Passthrough  PCopyVariant=Disabled  TRVariant=Disabled  FdbkBlocksVariant=Forward  IdealPFdbkVariant=Disabled  SatFdbkVariant=Disabled  DerivativeFilterVariant=Disabled  NVariant=Disabled  NCopyVariant=Disabled_SignalSpec  FilterICVariant=Disabled  IntegratorICVariant=InternalICs  ExternalResetVariant=Disabled  TRSumVariant=Passthrough  SumFdbkVariant=Disabled  SumVariant=Sum_PI
  Gain : Gain  Gain=D2
  Gain1 : Gain  Gain=D1
  Scope : Scope  NumInputPorts=2
  Sum : Sum  Inputs=|+-
  Sum1 : Sum  Inputs=|+-
  Sum2 : Sum  Inputs=|+-
  Out : Outport
  wires:
  Sum1/1 -> Discrete PID Controller/1
  Gain1/1 -> Scope/2, Sum1/2
  Discrete PID Controller/1 -> Sum/1
  Sum/1 -> Out/1
  Fd_dd/1 -> Gain/1
  Sum2/1 -> Discrete PID Controller1/1
  Gain/1 -> Sum/2
  Fd/1 -> Sum2/2
  Fd_d/1 -> Gain1/1
  Discrete PID Controller1/1 -> Scope/1, Sum1/1
  Demand/1 -> Sum2/1

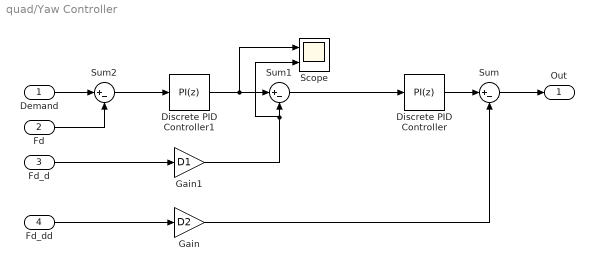
== system quad/Yaw Controller ==
  Demand : Inport
  Fd : Inport  Port=2
  Fd_d : Inport  Port=3
  Fd_dd : Inport  Port=4
  Discrete PID Controller : simulink/Continuous/PID Controller  Controller=PI  Form=Parallel  TimeDomain=Discrete-time  SampleTime=Ts  IntegratorMethod=Forward Euler  FilterMethod=Forward Euler  ControllerParametersSource=internal  P=P2  I=I2  D=0  UseFilter=off  N=100  TunerSelectOption=Transfer Function Based (PID Tuner App)  InitialConditionSource=internal  InitialConditionForIntegrator=0  InitialConditionForFilter=0  DifferentiatorICPrevScaledInput=0  ExternalReset=none  TrackingMode=off  Kt=1  LimitOutput=off  UpperSaturationLimit=inf  LowerSaturationLimit=-inf  LinearizeAsGain=off  AntiWindupMode=none  Kb=1  POutMin=[]  POutMax=[]  IOutMin=[]  IOutMax=[]  DOutMin=[]  DOutMax=[]  NOutMin=[]  NOutMax=[]  SumOutMin=[]  SumOutMax=[]  SaturationOutMin=[]  SaturationOutMax=[]  PParamMin=[]  PParamMax=[]  IParamMin=[]  IParamMax=[]  DParamMin=[]  DParamMax=[]  NParamMin=[]  NParamMax=[]  KbParamMin=[]  KbParamMax=[]  KtParamMin=[]  KtParamMax=[]  KbOutMin=[]  KbOutMax=[]  KtOutMin=[]  KtOutMax=[]  IntegratorOutMin=[]  IntegratorOutMax=[]  FilterOutMin=[]  FilterOutMax=[]  SumI1OutMin=[]  SumI1OutMax=[]  SumI2OutMin=[]  SumI2OutMax=[]  SumI3OutMin=[]  SumI3OutMax=[]  SumI4OutMin=[]  SumI4OutMax=[]  SumDOutMin=[]  SumDOutMax=[]  DifferentiatorOutMin=[]  DifferentiatorOutMax=[]  FilterDiffOutCoefMin=[]  FilterDiffOutCoefMax=[]  ReciprocalOutMin=[]  ReciprocalOutMax=[]  SumDenOutMin=[]  SumDenOutMax=[]  SumNumOutMin=[]  SumNumOutMax=[]  DivideOutMin=[]  DivideOutMax=[]  IntegratorContinuousStateAttributes=''  IntegratorStateMustResolveToSignalObject=off  IntegratorRTWStateStorageClass=Auto  FilterContinuousStateAttributes=''  FilterStateMustResolveToSignalObject=off  FilterRTWStateStorageClass=Auto  ParallelPVariant=InternalParameters  IdealPVariant=Disabled  IVariant=InternalParameters  DVariant=Disabled  IntegratorVariant=Discrete  SatVariant=Disabled  AWVariant=Passthrough  PCopyVariant=Disabled  TRVariant=Disabled  FdbkBlocksVariant=Forward  IdealPFdbkVariant=Disabled  SatFdbkVariant=Disabled  DerivativeFilterVariant=Disabled  NVariant=Disabled  NCopyVariant=Disabled_SignalSpec  FilterICVariant=Disabled  IntegratorICVariant=InternalICs  ExternalResetVariant=Disabled  TRSumVariant=Passthrough  SumFdbkVariant=Disabled  SumVariant=Sum_PI
  Discrete PID Controller1 : simulink/Continuous/PID Controller  Controller=PI  Form=Parallel  TimeDomain=Discrete-time  SampleTime=Ts  IntegratorMethod=Forward Euler  FilterMethod=Forward Euler  ControllerParametersSource=internal  P=P1  I=I1  D=0  UseFilter=off  N=100  TunerSelectOption=Transfer Function Based (PID Tuner App)  InitialConditionSource=internal  InitialConditionForIntegrator=0  InitialConditionForFilter=0  DifferentiatorICPrevScaledInput=0  ExternalReset=none  TrackingMode=off  Kt=1  LimitOutput=off  UpperSaturationLimit=inf  LowerSaturationLimit=-inf  LinearizeAsGain=off  AntiWindupMode=none  Kb=1  POutMin=[]  POutMax=[]  IOutMin=[]  IOutMax=[]  DOutMin=[]  DOutMax=[]  NOutMin=[]  NOutMax=[]  SumOutMin=[]  SumOutMax=[]  SaturationOutMin=[]  SaturationOutMax=[]  PParamMin=[]  PParamMax=[]  IParamMin=[]  IParamMax=[]  DParamMin=[]  DParamMax=[]  NParamMin=[]  NParamMax=[]  KbParamMin=[]  KbParamMax=[]  KtParamMin=[]  KtParamMax=[]  KbOutMin=[]  KbOutMax=[]  KtOutMin=[]  KtOutMax=[]  IntegratorOutMin=[]  IntegratorOutMax=[]  FilterOutMin=[]  FilterOutMax=[]  SumI1OutMin=[]  SumI1OutMax=[]  SumI2OutMin=[]  SumI2OutMax=[]  SumI3OutMin=[]  SumI3OutMax=[]  SumI4OutMin=[]  SumI4OutMax=[]  SumDOutMin=[]  SumDOutMax=[]  DifferentiatorOutMin=[]  DifferentiatorOutMax=[]  FilterDiffOutCoefMin=[]  FilterDiffOutCoefMax=[]  ReciprocalOutMin=[]  ReciprocalOutMax=[]  SumDenOutMin=[]  SumDenOutMax=[]  SumNumOutMin=[]  SumNumOutMax=[]  DivideOutMin=[]  DivideOutMax=[]  IntegratorContinuousStateAttributes=''  IntegratorStateMustResolveToSignalObject=off  IntegratorRTWStateStorageClass=Auto  FilterContinuousStateAttributes=''  FilterStateMustResolveToSignalObject=off  FilterRTWStateStorageClass=Auto  ParallelPVariant=InternalParameters  IdealPVariant=Disabled  IVariant=InternalParameters  DVariant=Disabled  IntegratorVariant=Discrete  SatVariant=Disabled  AWVariant=Passthrough  PCopyVariant=Disabled  TRVariant=Disabled  FdbkBlocksVariant=Forward  IdealPFdbkVariant=Disabled  SatFdbkVariant=Disabled  DerivativeFilterVariant=Disabled  NVariant=Disabled  NCopyVariant=Disabled_SignalSpec  FilterICVariant=Disabled  IntegratorICVariant=InternalICs  ExternalResetVariant=Disabled  TRSumVariant=Passthrough  SumFdbkVariant=Disabled  SumVariant=Sum_PI
  Gain : Gain  Gain=D2
  Gain1 : Gain  Gain=D1
  Scope : Scope  NumInputPorts=2
  Sum : Sum  Inputs=|+-
  Sum1 : Sum  Inputs=|+-
  Sum2 : Sum  Inputs=|+-
  Out : Outport
  wires:
  Demand/1 -> Sum2/1
  Discrete PID Controller1/1 -> Scope/1, Sum1/1
  Fd_d/1 -> Gain1/1
  Fd/1 -> Sum2/2
  Gain/1 -> Sum/2
  Sum2/1 -> Discrete PID Controller1/1
  Fd_dd/1 -> Gain/1
  Sum/1 -> Out/1
  Discrete PID Controller/1 -> Sum/1
  Gain1/1 -> Scope/2, Sum1/2
  Sum1/1 -> Discrete PID Controller/1

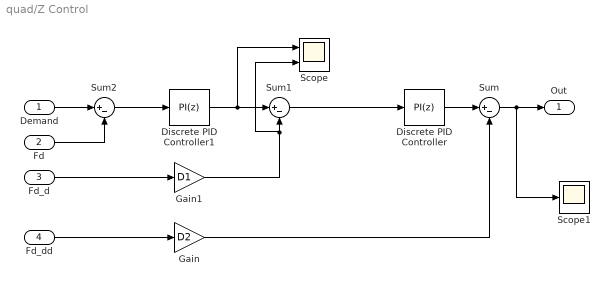
== system quad/Z Control ==
  Demand : Inport
  Fd : Inport  Port=2
  Fd_d : Inport  Port=3
  Fd_dd : Inport  Port=4
  Discrete PID Controller : simulink/Continuous/PID Controller  Controller=PI  Form=Parallel  TimeDomain=Discrete-time  SampleTime=Ts  IntegratorMethod=Forward Euler  FilterMethod=Forward Euler  ControllerParametersSource=internal  P=P2  I=I2  D=0  UseFilter=off  N=100  TunerSelectOption=Transfer Function Based (PID Tuner App)  InitialConditionSource=internal  InitialConditionForIntegrator=0  InitialConditionForFilter=0  DifferentiatorICPrevScaledInput=0  ExternalReset=none  TrackingMode=off  Kt=1  LimitOutput=off  UpperSaturationLimit=inf  LowerSaturationLimit=-inf  LinearizeAsGain=off  AntiWindupMode=none  Kb=1  POutMin=[]  POutMax=[]  IOutMin=[]  IOutMax=[]  DOutMin=[]  DOutMax=[]  NOutMin=[]  NOutMax=[]  SumOutMin=[]  SumOutMax=[]  SaturationOutMin=[]  SaturationOutMax=[]  PParamMin=[]  PParamMax=[]  IParamMin=[]  IParamMax=[]  DParamMin=[]  DParamMax=[]  NParamMin=[]  NParamMax=[]  KbParamMin=[]  KbParamMax=[]  KtParamMin=[]  KtParamMax=[]  KbOutMin=[]  KbOutMax=[]  KtOutMin=[]  KtOutMax=[]  IntegratorOutMin=[]  IntegratorOutMax=[]  FilterOutMin=[]  FilterOutMax=[]  SumI1OutMin=[]  SumI1OutMax=[]  SumI2OutMin=[]  SumI2OutMax=[]  SumI3OutMin=[]  SumI3OutMax=[]  SumI4OutMin=[]  SumI4OutMax=[]  SumDOutMin=[]  SumDOutMax=[]  DifferentiatorOutMin=[]  DifferentiatorOutMax=[]  FilterDiffOutCoefMin=[]  FilterDiffOutCoefMax=[]  ReciprocalOutMin=[]  ReciprocalOutMax=[]  SumDenOutMin=[]  SumDenOutMax=[]  SumNumOutMin=[]  SumNumOutMax=[]  DivideOutMin=[]  DivideOutMax=[]  IntegratorContinuousStateAttributes=''  IntegratorStateMustResolveToSignalObject=off  IntegratorRTWStateStorageClass=Auto  FilterContinuousStateAttributes=''  FilterStateMustResolveToSignalObject=off  FilterRTWStateStorageClass=Auto  ParallelPVariant=InternalParameters  IdealPVariant=Disabled  IVariant=InternalParameters  DVariant=Disabled  IntegratorVariant=Discrete  SatVariant=Disabled  AWVariant=Passthrough  PCopyVariant=Disabled  TRVariant=Disabled  FdbkBlocksVariant=Forward  IdealPFdbkVariant=Disabled  SatFdbkVariant=Disabled  DerivativeFilterVariant=Disabled  NVariant=Disabled  NCopyVariant=Disabled_SignalSpec  FilterICVariant=Disabled  IntegratorICVariant=InternalICs  ExternalResetVariant=Disabled  TRSumVariant=Passthrough  SumFdbkVariant=Disabled  SumVariant=Sum_PI
  Discrete PID Controller1 : simulink/Continuous/PID Controller  Controller=PI  Form=Parallel  TimeDomain=Discrete-time  SampleTime=Ts  IntegratorMethod=Forward Euler  FilterMethod=Forward Euler  ControllerParametersSource=internal  P=P1  I=I1  D=0  UseFilter=off  N=100  TunerSelectOption=Transfer Function Based (PID Tuner App)  InitialConditionSource=internal  InitialConditionForIntegrator=0  InitialConditionForFilter=0  DifferentiatorICPrevScaledInput=0  ExternalReset=none  TrackingMode=off  Kt=1  LimitOutput=off  UpperSaturationLimit=inf  LowerSaturationLimit=-inf  LinearizeAsGain=off  AntiWindupMode=none  Kb=1  POutMin=[]  POutMax=[]  IOutMin=[]  IOutMax=[]  DOutMin=[]  DOutMax=[]  NOutMin=[]  NOutMax=[]  SumOutMin=[]  SumOutMax=[]  SaturationOutMin=[]  SaturationOutMax=[]  PParamMin=[]  PParamMax=[]  IParamMin=[]  IParamMax=[]  DParamMin=[]  DParamMax=[]  NParamMin=[]  NParamMax=[]  KbParamMin=[]  KbParamMax=[]  KtParamMin=[]  KtParamMax=[]  KbOutMin=[]  KbOutMax=[]  KtOutMin=[]  KtOutMax=[]  IntegratorOutMin=[]  IntegratorOutMax=[]  FilterOutMin=[]  FilterOutMax=[]  SumI1OutMin=[]  SumI1OutMax=[]  SumI2OutMin=[]  SumI2OutMax=[]  SumI3OutMin=[]  SumI3OutMax=[]  SumI4OutMin=[]  SumI4OutMax=[]  SumDOutMin=[]  SumDOutMax=[]  DifferentiatorOutMin=[]  DifferentiatorOutMax=[]  FilterDiffOutCoefMin=[]  FilterDiffOutCoefMax=[]  ReciprocalOutMin=[]  ReciprocalOutMax=[]  SumDenOutMin=[]  SumDenOutMax=[]  SumNumOutMin=[]  SumNumOutMax=[]  DivideOutMin=[]  DivideOutMax=[]  IntegratorContinuousStateAttributes=''  IntegratorStateMustResolveToSignalObject=off  IntegratorRTWStateStorageClass=Auto  FilterContinuousStateAttributes=''  FilterStateMustResolveToSignalObject=off  FilterRTWStateStorageClass=Auto  ParallelPVariant=InternalParameters  IdealPVariant=Disabled  IVariant=InternalParameters  DVariant=Disabled  IntegratorVariant=Discrete  SatVariant=Disabled  AWVariant=Passthrough  PCopyVariant=Disabled  TRVariant=Disabled  FdbkBlocksVariant=Forward  IdealPFdbkVariant=Disabled  SatFdbkVariant=Disabled  DerivativeFilterVariant=Disabled  NVariant=Disabled  NCopyVariant=Disabled_SignalSpec  FilterICVariant=Disabled  IntegratorICVariant=InternalICs  ExternalResetVariant=Disabled  TRSumVariant=Passthrough  SumFdbkVariant=Disabled  SumVariant=Sum_PI
  Gain : Gain  Gain=D2
  Gain1 : Gain  Gain=D1
  Scope : Scope  NumInputPorts=2
  Scope1 : Scope
  Sum : Sum  Inputs=|+-
  Sum1 : Sum  Inputs=|+-
  Sum2 : Sum  Inputs=|+-
  Out : Outport
  wires:
  Gain1/1 -> Scope/2, Sum1/2
  Discrete PID Controller/1 -> Sum/1
  Sum/1 -> Scope1/1, Out/1
  Fd_dd/1 -> Gain/1
  Sum2/1 -> Discrete PID Controller1/1
  Gain/1 -> Sum/2
  Fd/1 -> Sum2/2
  Fd_d/1 -> Gain1/1
  Discrete PID Controller1/1 -> Scope/1, Sum1/1
  Demand/1 -> Sum2/1
  Sum1/1 -> Discrete PID Controller/1

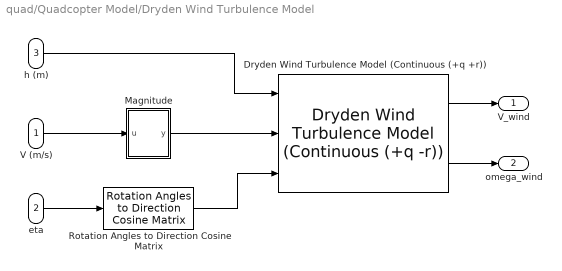
== system quad/Quadcopter Model/Dryden Wind Turbulence Model ==
  V (m/s) : Inport
  eta : Inport  Port=2
  h (m) : Inport  Port=3
  Dryden Wind Turbulence Model (Continuous (+q +r)) : aerolibwind2/Dryden Wind Turbulence Model  (Continuous (+q -r))  units=Metric (MKS)  spec=MIL-F-8785C  model=Discrete Dryden (+q +r)  W20=ws  Wdeg=0  TurbProb=2x10^-1  L_high=533.4  Wingspan=0.5  ts=0.1  Seed=[23345 23346 23347 23348]  T_on=on
      settings: SourceProductName=Aerospace Blockset
  Magnitude : MATLAB Function  TreatAsAtomicUnit=on
  Rotation Angles to Direction Cosine Matrix : sharedtransform/Rotation Angles to Direction Cosine Matrix  rotationOrder=XYZ  aMode=aMode
      settings: SourceProductBaseCode=AE
  V_wind : Outport
  omega_wind : Outport  Port=2
  wires:
  eta/1 -> Rotation Angles to Direction Cosine Matrix/1
  V (m/s)/1 -> Magnitude/1(u)
  Dryden Wind Turbulence Model (Continuous (+q +r))/2 -> omega_wind/1
  Dryden Wind Turbulence Model (Continuous (+q +r))/1 -> V_wind/1
  Rotation Angles to Direction Cosine Matrix/1 -> Dryden Wind Turbulence Model (Continuous (+q +r))/3
  Magnitude/1(y) -> Dryden Wind Turbulence Model (Continuous (+q +r))/2
  h (m)/1 -> Dryden Wind Turbulence Model (Continuous (+q +r))/1

== matlab function quad/Quadcopter Model/Omega Calculator ==
  data: P input; omega output; theta_d input double size=3
function omega = fcn(P, theta_d)
%#codegen

omega = P * theta_d;

== matlab function quad/Quadcopter Model/Angular Velocities ==
  data: W1 input; W2 input; W3 input; W4 input; x4_d output size=3; Ixx parameter; Iyy parameter; Izz parameter; k parameter; L parameter; b parameter; omega input size=3
function x4_d = fcn(W1, W2, W3, W4, Ixx, Iyy, Izz, k, L, b, omega)
%#codegen

%L = distance from center of mass to motor
%k = relationship between torque and motor speed squared



% Motor Torques in pitch roll and yaw directions
tor_b = [L * k * (W1^2 - W3^2);
         L * k * (W2^2 - W4^2);
         b * (W1^2 - W2^2 + W3^2 - W4^2)];
     
% Inertial matrix
I = [Ixx, 0,   0;
     0,   Iyy, 0;
     0,   0,   Izz];

% Euler's rigid body dynamics equation
x4_d = I\(tor_b - cross(omega, (I*omega)) );

== matlab function quad/Quadcopter Model/Angular Displacement ==
  data: x4 input size=3; P input; x3_d output
function x3_d = fcn(x4, P)
%#codegen

x3_d = P\x4;

== matlab function quad/Quadcopter Model/P ==
  data: omega input size=3; P output
function P = fcn(omega)

P = [1,  0,              -sin(omega(2)); 
     0,  cos(omega(1)),  cos(omega(2)) * sin(omega(1)); 
     0, -sin(omega(1)),  cos(omega(2)) * cos(omega(1))];

== matlab function quad/Quadcopter Model/ZYZ Euler Angles ==
  data: omega input size=3; R output
function R = fcn(omega)
%#codegen

a = omega(1);
b = omega(2);
c = omega(3);

R = [cos(c)*cos(b), cos(c)*sin(b)*sin(c) - sin(c)*cos(a),...
     cos(c)*sin(b)*cos(a) + sin(c)*sin(a);
     sin(c)*cos(b), sin(c)*sin(b)*sin(a) + cos(c)*cos(a)...
     sin(c)*sin(b)*cos(a) - cos(c)*sin(a);
     -sin(b), cos(b)*sin(a), cos(b)*cos(a)];

== matlab function quad/Quadcopter Model/Thrust ==
  data: W1 input; T_b output; W2 input; W3 input; W4 input; k parameter
function T_b = fcn(W1, W2, W3, W4, k)
%#codegen
T_b =[0; 0; k * (W1^2 + W2^2 + W3^2 + W4^2)];

== matlab function quad/Quadcopter Model/Fluid Friction ==
  data: velocity input size=3; F_d output size=3; Ax parameter; Ay parameter; Az parameter
function F_d = fcn(velocity, Ax, Ay, Az)
%#codegen

A = diag([Ax Ay Az]);

F_d = A * velocity;

== matlab function quad/Quadcopter Model/Linear Velocity ==
  data: R input; x2_d output size=3; T_b input size=3; F_d input size=3; g parameter; m parameter
function x2_d = fcn(R, T_b, F_d, g, m)
%#codegen
g_vec = [0; 0; -g];

x2_d = g_vec + (1/m) * R * T_b - (1/m) * F_d;

== matlab function quad/Quadcopter Model/Dryden Wind Turbulence Model/Magnitude ==
  data: u input size=3; y output size=1
function y = fcn(u)
%#codegen

y = sqrt(u' * u);
